simulink library "FlowRate"  (R2024a)
settings: Solver=VariableStepAuto  StartTime=0.0  StopTime=10.0  RelTol=1e-3
undefined symbols (not defined in the file): raptor_xcp_function, StateSignal
libraries: Utilities x4, simulink x4, Raptor_lib x4
settings Model: Creator=serga  LastModifiedBy=serga

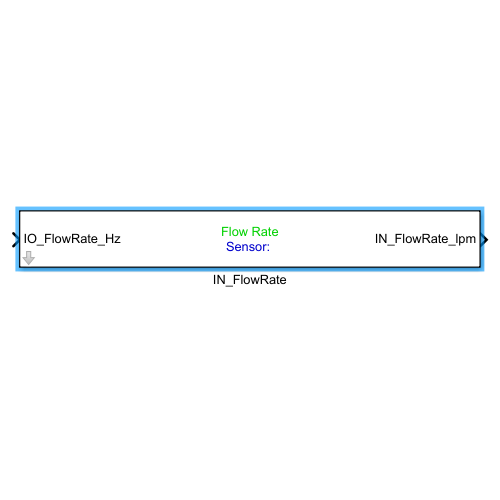
[thumbnail: Simulink's stored preview of the top-level diagram]
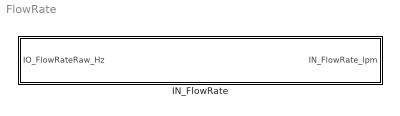
== system FlowRate ==
  IN_FlowRate : Subsystem  mask{pos=''}
      mask prompts: pos "Position"
      mask Display:
      | color('green')
      | disp('Flow Rate\n');
      | color('blue')
      | disp(['\nSensor: ' pos]);
      | color('black')
      | port_label('input', 1, ['IO_FlowRate' pos '_Hz']);
      | port_label('output', 1, ['IN_FlowRate' pos '_lpm']);

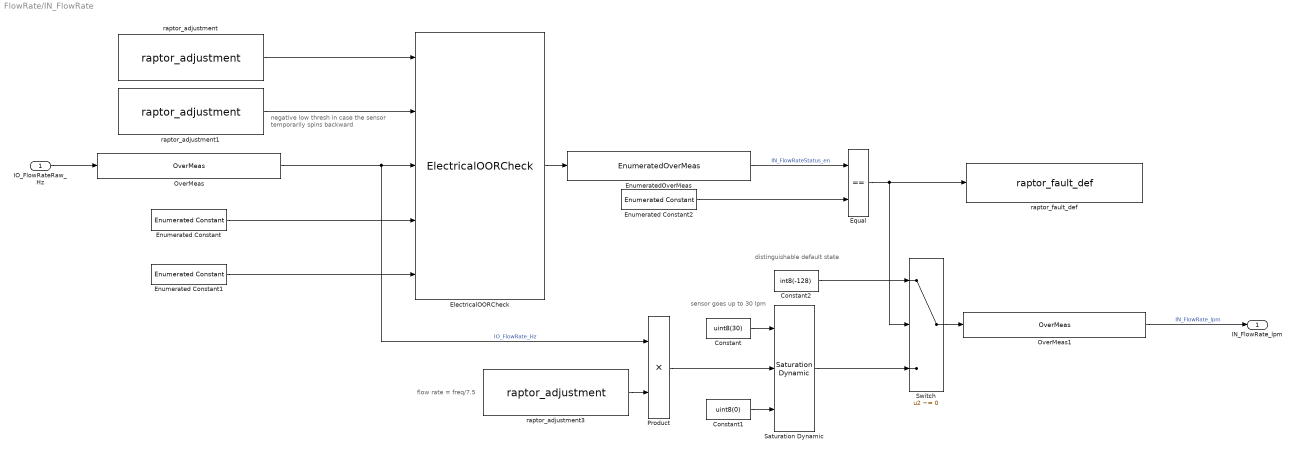
== system FlowRate/IN_FlowRate ==
  note: distinguishable default state
  note: sensor goes up to 30 lpm
  note: flow rate = freq/7.5
  note: negative low thresh in case the sensor temporarily spins backward
  IO_FlowRateRaw_Hz : Inport
  Constant : Constant  Value=uint8(30)
  Constant1 : Constant  Value=uint8(0)
  Constant2 : Constant  Value=int8(-128)
  ElectricalOORCheck : Utilities/ElectricalOORCheck
  Enumerated Constant : simulink/Sources/Enumerated Constant  OutDataTypeStr=Enum: StateSignal  Value=StateSignal.Normal  SampleTime=inf
  Enumerated Constant1 : simulink/Sources/Enumerated Constant  OutDataTypeStr=Enum: StateSignal  Value=StateSignal.Fault  SampleTime=inf
  Enumerated Constant2 : simulink/Sources/Enumerated Constant  OutDataTypeStr=Enum: StateSignal  Value=StateSignal.Fault  SampleTime=inf
  EnumeratedOverMeas : Utilities/EnumeratedOverMeas  sigName=['IN_FlowRate' pos 'Status_en']  enumName='StateSignal'
  Equal : RelationalOperator  Operator===  OutDataTypeStr=boolean  RndMeth=Simplest  InputSameDT=off
  OverMeas : Utilities/OverMeas  sigName=['IO_FlowRate' pos '_Hz']  minimum=-inf  maximum=inf
  OverMeas1 : Utilities/OverMeas  sigName=['IN_FlowRate' pos '_lpm']  minimum=0  maximum=100
  Product : Product
  Saturation Dynamic : simulink/Discontinuities/Saturation Dynamic  OutMin=[]  OutMax=[]  OutDataTypeStr=Inherit: Same as second input  OutDataType=fixdt(1, 16)  OutScaling=2^-10  DoSatur=off
  Switch : Switch  Criteria=u2 ~= 0  SaturateOnIntegerOverflow=off  InputSameDT=off
  raptor_adjustment : Raptor_lib/Data Storage/raptor_adjustment  paramName=['IN_FlowRate' pos 'HighThresh_Hz']  nameSource=Parameter  initValue=225  dataType=single  storage=Calibration  calDispType=Number  calEnum={'False', 'True'}  calGain=1.0  calOffset=0.0  calMax=5  calMin=0  calFormat='-1'  calUnit=''  calHelp=''  calAccess=1  calFunction=raptor_xcp_function(gcb)  calDispHeaders=off  calColHeaders={'Col1' 'Col2' 'Col3'}  calRowHeaders={'Row1' 'Row2' 'Row3'}
      settings: SourceProductName=Raptor
  raptor_adjustment1 : Raptor_lib/Data Storage/raptor_adjustment  paramName=['IN_FlowRate' pos 'LowThresh_V']  nameSource=Parameter  initValue=-5  dataType=single  storage=Calibration  calDispType=Number  calEnum={'False', 'True'}  calGain=1.0  calOffset=0.0  calMax=5  calMin=0  calFormat='-1'  calUnit=''  calHelp=''  calAccess=1  calFunction=raptor_xcp_function(gcb)  calDispHeaders=off  calColHeaders={'Col1' 'Col2' 'Col3'}  calRowHeaders={'Row1' 'Row2' 'Row3'}
      settings: SourceProductName=Raptor
  raptor_adjustment3 : Raptor_lib/Data Storage/raptor_adjustment  paramName=['IN_FlowRate' pos 'Scale_na']  nameSource=Parameter  initValue=1/7.5  dataType=single  storage=Calibration  calDispType=Number  calEnum={'False', 'True'}  calGain=1.0  calOffset=0.0  calMax=5  calMin=0  calFormat='-1'  calUnit=''  calHelp=''  calAccess=1  calFunction=raptor_xcp_function(gcb)  calDispHeaders=off  calColHeaders={'Col1' 'Col2' 'Col3'}  calRowHeaders={'Row1' 'Row2' 'Row3'}
      settings: SourceProductName=Raptor
  raptor_fault_def : Raptor_lib/Faults/raptor_fault_def  faultName=['IN_FlowRate' pos 'Fault']  persist=off  sticky=off  emisRelated=off  singleTrip=off  clearMethod=Standard  xLimit=25  yLimit=50  calEnable=on  addDisable=off  calAccess=1  calFunction='System | FaultManager'
      settings: SourceProductName=Raptor
  IN_FlowRate_lpm : Outport
  wires:
  Switch/1 -> OverMeas1/1
  OverMeas1/1 -> IN_FlowRate_lpm/1  "IN_FlowRate_lpm"
  Constant2/1 -> Switch/1
  Constant1/1 -> Saturation Dynamic/3
  Constant/1 -> Saturation Dynamic/1
  Saturation Dynamic/1 -> Switch/3
  raptor_adjustment3/1 -> Product/2
  EnumeratedOverMeas/1 -> Equal/1  "IN_FlowRateStatus_en"
  Equal/1 -> raptor_fault_def/1, Switch/2
  Enumerated Constant2/1 -> Equal/2
  ElectricalOORCheck/1 -> EnumeratedOverMeas/1
  Enumerated Constant1/1 -> ElectricalOORCheck/5
  Enumerated Constant/1 -> ElectricalOORCheck/4
  raptor_adjustment1/1 -> ElectricalOORCheck/2
  raptor_adjustment/1 -> ElectricalOORCheck/1
  OverMeas/1 -> Product/1, ElectricalOORCheck/3  "IO_FlowRate_Hz"
  IO_FlowRateRaw_Hz/1 -> OverMeas/1
  Product/1 -> Saturation Dynamic/2
